simulink model "LQG_kalman"  (R2025a)
settings: Solver=VariableStepAuto  StartTime=0.0  StopTime=inf  RelTol=1e-3
undefined symbols (not defined in the file): A, Ad, Ad_c, Aobs, Aobs_d, B, Bd, Bd_c, Bobs, Bobs_d, C, Cd, Cd_c, Cobs, Cobs_d, D, Dd, Dd_c, Dobs, Dobs_d, G, Gd, Ts, x, y, z
libraries: ros2lib x2
settings Model: Creator=Sandro  LastModifiedBy=Sandro

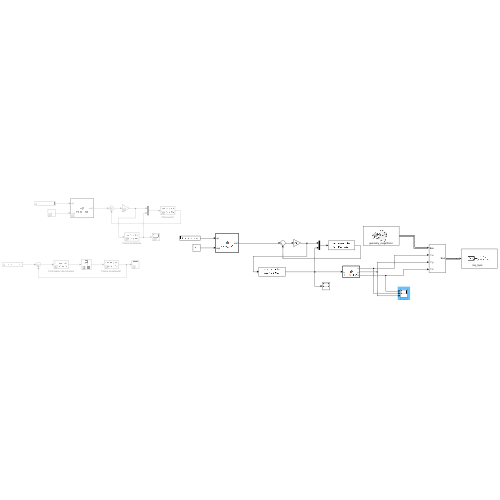
[thumbnail: Simulink's stored preview of the top-level diagram]
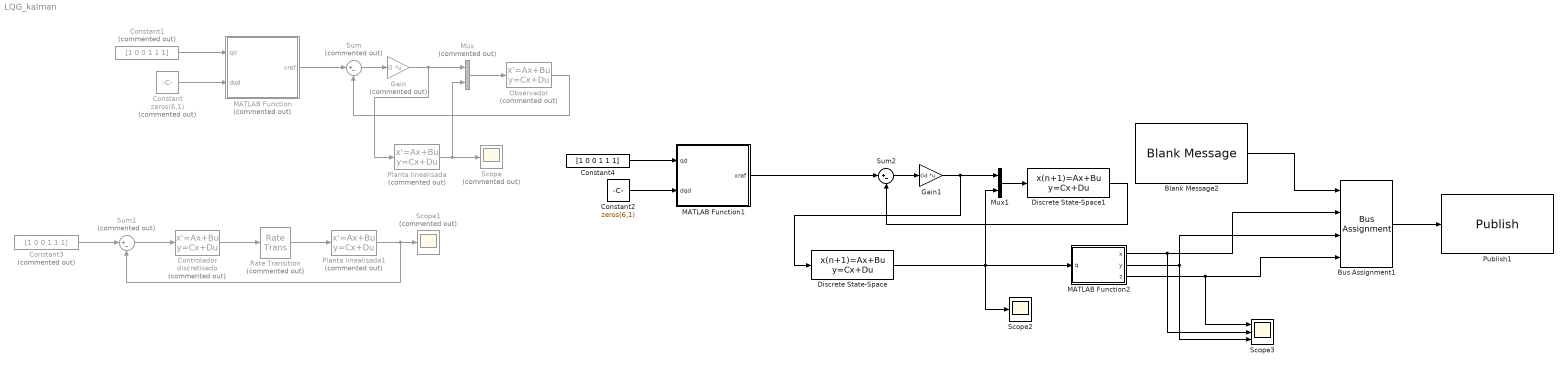
== system LQG_kalman ==
  Blank Message2 : ros2lib/Blank Message  messageClass=Message  entityType=geometry_msgs/Point  messageType=geometry_msgs/Point  SampleTime=inf
  Bus Assignment1 : BusAssignment  AssignedSignals=x,y,z
  Constant : Constant  Commented=on  Value=zeros(6,1)
  Constant1 : Constant  Commented=on  Value=[1 0 0 1 1 1]
  Constant2 : Constant  Value=zeros(6,1)
  Constant3 : Constant  Commented=on  Value=[1 0 0 1 1 1]
  Constant4 : Constant  Value=[1 0 0 1 1 1]
  Controlador discretisado : StateSpace  Commented=on  A=Ad_c  B=Bd_c  C=Cd_c  D=Dd_c  InitialCondition=0
  Discrete State-Space : DiscreteStateSpace  A=Ad  B=Bd  C=Cd  D=Dd  SampleTime=Ts
  Discrete State-Space1 : DiscreteStateSpace  A=Aobs_d  B=Bobs_d  C=Cobs_d  D=Dobs_d  SampleTime=Ts
  Gain : Gain  Commented=on  Gain=G  Multiplication=Matrix(K*u)
  Gain1 : Gain  Gain=Gd  Multiplication=Matrix(K*u)
  MATLAB Function : MATLAB Function  Commented=on  TreatAsAtomicUnit=on
  MATLAB Function1 : MATLAB Function  TreatAsAtomicUnit=on
  MATLAB Function2 : MATLAB Function  TreatAsAtomicUnit=on
  Mux : Mux  Commented=on  Inputs=2
  Mux1 : Mux  Inputs=2
  Observador : StateSpace  Commented=on  A=Aobs  B=Bobs  C=Cobs  D=Dobs  InitialCondition=0
  Planta linealisada : StateSpace  Commented=on  A=A  B=B  C=C  D=D  InitialCondition=0
  Planta linealisada1 : StateSpace  Commented=on  A=Ad  B=Bd  C=Cd  D=Dd  InitialCondition=0
  Publish1 : ros2lib/Publish  topicSource=Specify your own  topic=/my_topic  messageType=geometry_msgs/Point  QOSHistory=Keep last  QOSDepth=10  QOSReliability=Reliable  QOSDurability=Volatile  QOSDeadline=Inf  QOSLifespan=Inf  QOSLiveliness=Automatic  QOSLeaseDuration=Inf  QOSAvoidROSNamespaceConventions=off
  Rate Transition : RateTransition  Commented=on  OutPortSampleTime=Ts
  Scope : Scope  Commented=on
      settings: ActiveDisplayYMinimum=-0.13865212313210939  ActiveDisplayYMaximum=0.50074348198893537
  Scope1 : Scope  Commented=on
      settings: ActiveDisplayYMinimum=-503.36541572061844  ActiveDisplayYMaximum=137.5253415074734
  Scope2 : Scope
      settings: ActiveDisplayYMinimum=-0.2915540002198872  ActiveDisplayYMaximum=1.1809744489877028  DataLoggingVariableName=ScopeData2
  Scope3 : Scope  NumInputPorts=3
      settings: ActiveDisplayYMinimum=-0.66636319370533381  ActiveDisplayYMaximum=1.0681169371309323  DataLoggingVariableName=ScopeData3
  Sum : Sum  Commented=on  Inputs=|+-
  Sum1 : Sum  Commented=on  Inputs=|+-
  Sum2 : Sum  Inputs=|+-
  wires:
  Mux/1 -> Observador/1
  Gain/1 -> Planta linealisada/1, Mux/1
  Constant/1 -> MATLAB Function/2(dqd)
  Constant1/1 -> MATLAB Function/1(qd)
  Planta linealisada/1 -> Mux/2, Scope/1
  MATLAB Function/1(xref) -> Sum/1
  Sum/1 -> Gain/1
  Observador/1 -> Sum/2
  Controlador discretisado/1 -> Rate Transition/1
  Rate Transition/1 -> Planta linealisada1/1
  Sum1/1 -> Controlador discretisado/1
  Constant3/1 -> Sum1/1
  Planta linealisada1/1 -> Sum1/2, Scope1/1
  Constant2/1 -> MATLAB Function1/2(dqd)
  Sum2/1 -> Gain1/1
  Constant4/1 -> MATLAB Function1/1(qd)
  MATLAB Function1/1(xref) -> Sum2/1
  Discrete State-Space1/1 -> Sum2/2
  Discrete State-Space/1 -> MATLAB Function2/1(q), Mux1/2, Scope2/1
  Mux1/1 -> Discrete State-Space1/1
  Gain1/1 -> Discrete State-Space/1, Mux1/1
  MATLAB Function2/1(x) -> Scope3/2, Bus Assignment1/2
  MATLAB Function2/3(z) -> Scope3/1, Bus Assignment1/4
  Bus Assignment1/1 -> Publish1/1
  MATLAB Function2/2(y) -> Scope3/3, Bus Assignment1/3
  Blank Message2/1 -> Bus Assignment1/1

== matlab function LQG_kalman/MATLAB Function ==
  data: qd input; xref output; dqd input
function xref = make_xref(qd, dqd)
% make_xref  Devuelve x_ref = [qd; dqd] (12x1) para 6 DOF
% Entradas:
%  qd  - posicion deseada (6x1)
%  dqd - velocidad deseada (6x1) (opcional; si no se entrega se usa cero)
%
% Salida:
%  xref - referencia de estado 12x1 = [qd; dqd]

% Si no se suministra dqd, asumir ceros
if nargin < 2 || isempty(dqd)
    dqd = zeros(6,1);
end

% Asegurar columna
qd  = qd(:);
dqd = dqd(:);

% Validar tamaño
if numel(qd) ~= 6 || numel(dqd) ~= 6
    error('qd y dqd deben ser vectores de 6 elementos (6x1).');
end

% Construir xref
xref = [qd; dqd];

end

== matlab function LQG_kalman/MATLAB Function2 ==
  data: x output; q input; y output; z output
function [x, y, z] = FK_CRX5iA(q)
%#codegen

% q : vector 6x1 (radianes)

    % ===== 1. TABLA DH OFICIAL FANUC CRX-5iA =====
    DH = [
        0       pi/2     0.424     q(1);
        0.450   0        0         q(2);
        0.350   0        0         q(3);
        0       pi/2     0.420     q(4);
        0      -pi/2     0         q(5);
        0       0        0.080     q(6)
    ];

    % ===== 2. MATRIZ DE TRANSFORMACIÓN TOTAL =====
    T = eye(4);

    for i = 1:6
        a = DH(i,1);
        alpha = DH(i,2);
        d = DH(i,3);
        theta = DH(i,4);

        % Matriz Ai según DH estándar
        A = [...
            cos(theta),  -sin(theta)*cos(alpha),   sin(theta)*sin(alpha),   a*cos(theta); 
            sin(theta),   cos(theta)*cos(alpha),  -cos(theta)*sin(alpha),   a*sin(theta);
            0,            sin(alpha),              cos(alpha),              d;
            0,            0,                       0,                       1];

        T = T * A;
    end

    % ===== 3. POSICIÓN =====
    x = T(1,4);
    y = T(2,4);
    z = T(3,4);
end

== matlab function LQG_kalman/MATLAB Function1 ==
  data: qd input; xref output; dqd input
function xref = make_xref(qd, dqd)
% make_xref  Devuelve x_ref = [qd; dqd] (12x1) para 6 DOF
% Entradas:
%  qd  - posicion deseada (6x1)
%  dqd - velocidad deseada (6x1) (opcional; si no se entrega se usa cero)
%
% Salida:
%  xref - referencia de estado 12x1 = [qd; dqd]

% Si no se suministra dqd, asumir ceros
if nargin < 2 || isempty(dqd)
    dqd = zeros(6,1);
end

% Asegurar columna
qd  = qd(:);
dqd = dqd(:);

% Validar tamaño
if numel(qd) ~= 6 || numel(dqd) ~= 6
    error('qd y dqd deben ser vectores de 6 elementos (6x1).');
end

% Construir xref
xref = [qd; dqd];

end
